simulink library "uavsimBlockset_UAV3DVisualization"  (Simulink 8.6)
settings: Solver=ode45  StartTime=0.0  StopTime=10.0  RelTol=1e-3
undefined symbols (not defined in the file): uavsim
libraries: aerolibtransform2 x1, uavsimBlockset_UAV3DInterface x1
settings Model: Creator=mstolle  LastModifiedBy=j.bolting

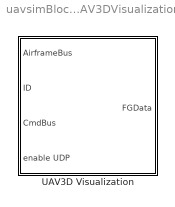
== system uavsimBlockset_UAV3DVisualization ==
  UAV3D Visualization : Subsystem  TreatAsAtomicUnit=on  SystemSampleTime=uavsim.simConfig.tsample_UAV3D  mask{mask_visual=2}
      mask prompts: mask_visual "3D model"
      mask TypeOptions mask_visual: 0 | 1 | 2 | 3

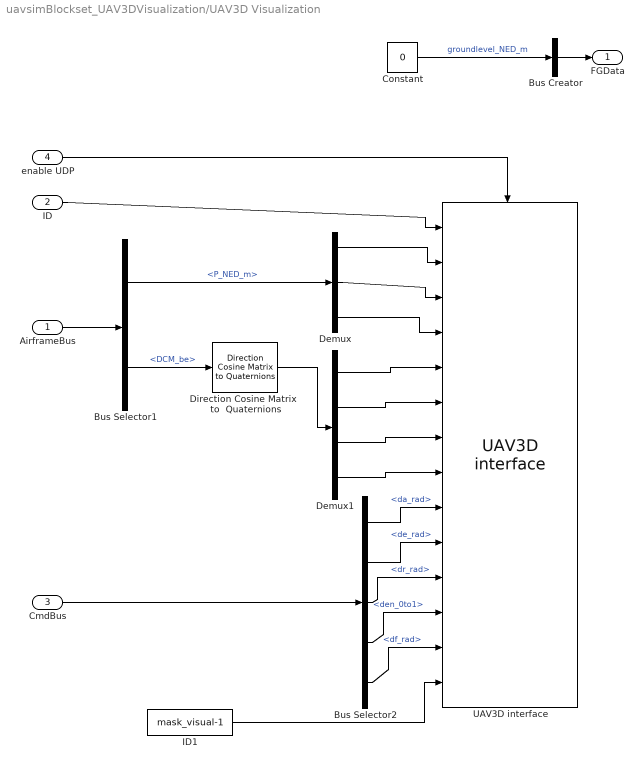
== system uavsimBlockset_UAV3DVisualization/UAV3D Visualization ==
  AirframeBus : Inport  OutDataTypeStr=Bus: Airframe
  ID : Inport  Port=2
  CmdBus : Inport  Port=3  OutDataTypeStr=Bus: CMD
  enable UDP : Inport  Port=4
  Bus Selector1 : BusSelector  OutputSignals=Kinematics.Position.P_NED_m,Kinematics.Attitude.DCM_be
  Bus Selector2 : BusSelector  OutputSignals=da_rad,de_rad,dr_rad,den_0to1,df_rad
  Bus Creator : BusCreator  Inputs=1  OutDataTypeStr=Bus: FlightGearData
  Constant : Constant  Value=0
  Demux : Demux  Outputs=3
  Demux1 : Demux
  Direction Cosine Matrix   to  Quaternions : aerolibtransform2/Direction Cosine Matrix  to Quaternions
  ID1 : Constant  Value=mask_visual-1
  UAV3D interface : uavsimBlockset_UAV3DInterface/UAV3D interface  ip='localhost'  udpport=4445
  FGData : Outport  OutDataTypeStr=Bus: FlightGearData
  wires:
  enable UDP/1 -> UAV3D interface/Enable
  ID1/1 -> UAV3D interface/14
  ID/1 -> UAV3D interface/1
  Direction Cosine Matrix   to  Quaternions/1 -> Demux1/1
  Demux1/4 -> UAV3D interface/8
  Demux1/3 -> UAV3D interface/7
  Demux1/2 -> UAV3D interface/6
  Demux1/1 -> UAV3D interface/5
  Bus Selector1/2 -> Direction Cosine Matrix   to  Quaternions/1  "<DCM_be>"
  Demux/1 -> UAV3D interface/2
  Demux/2 -> UAV3D interface/3
  Demux/3 -> UAV3D interface/4
  Bus Selector1/1 -> Demux/1  "<P_NED_m>"
  AirframeBus/1 -> Bus Selector1/1
  Constant/1 -> Bus Creator/1  "groundlevel_NED_m"
  Bus Creator/1 -> FGData/1
  CmdBus/1 -> Bus Selector2/1
  Bus Selector2/1 -> UAV3D interface/9  "<da_rad>"
  Bus Selector2/2 -> UAV3D interface/10  "<de_rad>"
  Bus Selector2/3 -> UAV3D interface/11  "<dr_rad>"
  Bus Selector2/4 -> UAV3D interface/12  "<den_0to1>"
  Bus Selector2/5 -> UAV3D interface/13  "<df_rad>"
